simulink model "JenaFox_NCm"  (R2022a)
settings: Solver=VariableStepAuto  StartTime=0.0  StopTime=terminationConditions.stopTime  FixedStep=0.0001  MaxStep=solverParams.maxStep  RelTol=solverParams.relTol  AbsTol=solverParams.absTol
undefined symbols (not defined in the file): amplifier, c_coupling, d_coupling, g, GC, GM_h, IC, IC_v, motorHip, motorKnee, mu, offset, prop_const, smiData, terminationConditions, v, X, Y, Z
libraries: sm_lib x51, nesl_utility x46, simulink x23, simulink_extras x12, dspswit3 x2
(part 3 of 4)

== system JenaFox_NCm/JenaFox Model/Knee_r ==
  Right torque : Inport
  PS-Simulink Converter1 : nesl_utility/PS-Simulink Converter  PhysicalDomain=network_engine_domain  SubClassName=ps_output  LeftPortType=input  RightPortType=output  PseudoPeriodic=off  Frequencies=[]  VectorFormat=1-D array  Unit=1  AffineConversion=off
      settings: SourceProductBaseCode=SS,PW,VE
  PS-Simulink Converter2 : nesl_utility/PS-Simulink Converter  PhysicalDomain=network_engine_domain  SubClassName=ps_output  LeftPortType=input  RightPortType=output  PseudoPeriodic=off  Frequencies=[]  VectorFormat=1-D array  Unit=1  AffineConversion=off
      settings: SourceProductBaseCode=SS,PW,VE
  PS-Simulink Converter3 : nesl_utility/PS-Simulink Converter  PhysicalDomain=network_engine_domain  SubClassName=ps_output  LeftPortType=input  RightPortType=output  PseudoPeriodic=off  Frequencies=[]  VectorFormat=1-D array  Unit=1  AffineConversion=off
      settings: SourceProductBaseCode=SS,PW,VE
  Simulink-PS Converter : nesl_utility/Simulink-PS Converter  PhysicalDomain=network_engine_domain  SubClassName=ps_input  LeftPortType=input  RightPortType=output  PseudoPeriodic=off  Frequencies=[]  NoiseDistribution=none  NoiseParameters=[]  Unit=1  AffineConversion=off  FilteringAndDerivatives=provide  SimscapeFilterOrder=1  InputFilterTimeConstant=0.001  UdotUserProvided=0
      settings: SourceProductBaseCode=SS,PW,VE
  knee_r : sm_lib/Joints/Revolute Joint  JointMode=Normal  SenseConstraintForce=off  SenseConstraintForceX=off  SenseConstraintForceY=off  SenseConstraintForceZ=off  SenseConstraintTorque=off  SenseConstraintTorqueX=off  SenseConstraintTorqueY=off  SenseConstraintTorqueZ=off  SenseTotalForce=off  SenseTotalForceX=off  SenseTotalForceY=off  SenseTotalForceZ=off  SenseTotalTorque=off  SenseTotalTorqueX=off  SenseTotalTorqueY=off  SenseTotalTorqueZ=off  CompositeWrenchDir=FollowerOnBase  CompositeWrenchFrame=BaseFrame  EquilibriumPosition=0  EquilibriumPositionUnits=rad  SpringStiffness=0  SpringStiffnessUnits=N*m/rad  DampingCoefficient=d_joint  DampingCoefficientUnits=N*m/(rad/s)  TorqueActuationMode=InputTorque  MotionActuationMode=ComputedMotion  SensePosition=on  SenseVelocity=on  SenseAcceleration=on  SenseTorqueForce=off  SenseLowerLimitTorqueForce=off  SenseUpperLimitTorqueForce=off  LowerLimitSpecify=on  LowerLimitBound=IC.limit.phi_knee  LowerLimitBoundUnits=rad  LowerLimitStiffness=c_hs  LowerLimitStiffnessUnits=N*m/deg  LowerLimitDamping=d_hs  LowerLimitDampingUnits=N*m/(deg/s)  LowerLimitTransitionRegionWidth=0.1  LowerLimitTransitionRegionWidthUnits=deg  UpperLimitSpecify=on  UpperLimitBound=0  UpperLimitBoundUnits=rad  UpperLimitStiffness=c_hs  UpperLimitStiffnessUnits=N*m/deg  UpperLimitDamping=d_hs  UpperLimitDampingUnits=N*m/(deg/s)  UpperLimitTransitionRegionWidth=0.1  UpperLimitTransitionRegionWidthUnits=deg  PositionTargetSpecify=on  PositionTargetPriority=High  PositionTargetValue=IC.phi.knee_r  PositionTargetValueUnits=rad  VelocityTargetSpecify=on  VelocityTargetPriority=High  VelocityTargetValue=IC.vphi.knee_r  VelocityTargetValueUnits=rad/s
  Thigh : PMIOPort  Side=Left
  Shank : PMIOPort  Port=2  Side=Right
  tag scope: aphi_knee_r=global, phi_knee_r=global, vphi_knee_r=global
  wires:
  Right torque/1 -> Simulink-PS Converter/1  "torque servo right"
  PS-Simulink Converter2/1 -> [phi_knee_r]
  PS-Simulink Converter3/1 -> [aphi_knee_r]
  PS-Simulink Converter1/1 -> [vphi_knee_r]
  connections:
  Simulink-PS Converter/RConn1 -- knee_r/LConn2
  knee_r/RConn1 -- Shank/RConn1
  PS-Simulink Converter2/LConn1 -- knee_r/RConn2
  knee_r/RConn3 -- PS-Simulink Converter1/LConn1
  knee_r/LConn1 -- Thigh/RConn1
  PS-Simulink Converter3/LConn1 -- knee_r/RConn4

== system JenaFox_NCm/JenaFox Model/Shank_bottom_l ==
  Rigid Transform : sm_lib/Frames and Transforms/Rigid Transform  TranslationMethod=None  TranslationStandardOffset=0  TranslationLengthUnit=m  TranslationStandardAxis=+Z  TranslationCartesianOffset=[0 0 0]  TranslationROffset=0  TranslationROffsetUnits=m  TranslationZOffset=0  TranslationZOffsetUnits=m  TranslationThetaOffset=0  TranslationThetaOffsetUnits=deg  RotationMethod=AlignedAxes  RotationAngleUnits=deg  RotationStandardAxis=+Z  RotationAngle=0.0  RotationArbitraryAxis=[0 0 1]  FollAlignAxisA=+X  BaseAlignAxisA=-X  FollAlignAxisB=+Z  BaseAlignAxisB=+Y  RotationSequenceAxes=FollowerAxes  RotationSequence=XYX  RotationSequenceAngles=[0 0 0]  RotationSequenceAnglesUnits=deg  RotationMatrix=[1 0 0; 0 1 0; 0 0 1]
  Solid : sm_lib/Body Elements/File Solid  ExtGeomFileName=shank_bottom_ipt_92530788.STEP  UnitType=FromFile  ExtGeomFileUnits=m  StepReaderType=OCC  ExportConvexHullGeometry=off  InertiaType=Custom  Mass=smiData.Solid(4).mass  MassUnits=kg  CenterOfMass=smiData.Solid(4).CoM  CenterOfMassUnits=mm  MomentsOfInertia=smiData.Solid(4).MoI  MomentsOfInertiaUnits=kg*mm^2  ProductsOfInertia=smiData.Solid(4).PoI  ProductsOfInertiaUnits=kg*mm^2  BasedOnType=Density  Density=1000  DensityUnits=kg/m^3  DoExposeReferenceFrame=on  SerializedFrames=<Frames><Frame><Id>Frame1</Id><Value><Name>ground_contact</Name><Origin><Source>GeometricFeature</Source><FeatureName>circular curve 105</FeatureName></Origin><PrimaryAxis><DefinedDirection>+Y</DefinedDirection><Source>ReferenceFrame</Source><SourceDirection>-Y</SourceDirection><FeatureName></FeatureName></PrimaryAxis><SecondaryAxis><DefinedDirection>+X</DefinedDirection><Source>ReferenceFrame</Source><SourceDirection>+X</SourceDirection><FeatureName></FeatureName></SecondaryAxis></Value></Frame><Frame><Id>Frame2</Id><Value><Name>spring_bottom</Name><Origin><Source>GeometricFeature</Source><FeatureName>circular curve 81</FeatureName></Origin><PrimaryAxis><DefinedDirection>+Y</DefinedDirection><Source>ReferenceFrame</Source><SourceDirection>-Y</SourceDirection><FeatureName></FeatureName></PrimaryAxis><SecondaryAxis><DefinedDirection>+X</DefinedDirection><Source>ReferenceFrame</Source><SourceDirection>+X</SourceDirection><FeatureName></FeatureName></SecondaryAxis></Value></Frame></Frames>  GraphicType=FromGeometry  MarkerShape=Sphere  MarkerSize=10  GraphicVisPropType=SimpleVisualProperties  GraphicDiffuseColor=smiData.Solid(4).color  GraphicSpecularColor=[0.5 0.5 0.5 1.0]  GraphicAmbientColor=[0.15 0.15 0.15 1.0]  GraphicEmissiveColor=[0.0 0.0 0.0 1.0]  GraphicShininess=75  GraphicOpacity=smiData.Solid(4).opacity
  Linear elastic joint : PMIOPort  Side=Left
  Toe : PMIOPort  Port=2  Side=Right
  connections:
  Toe/RConn1 -- Solid/LConn1
  Rigid Transform/RConn1 -- Linear elastic joint/RConn1
  Rigid Transform/LConn1 -- Solid/LConn2

== system JenaFox_NCm/JenaFox Model/Shank_bottom_r ==
  Rigid Transform : sm_lib/Frames and Transforms/Rigid Transform  TranslationMethod=None  TranslationStandardOffset=0  TranslationLengthUnit=m  TranslationStandardAxis=+Z  TranslationCartesianOffset=[0 0 0]  TranslationROffset=0  TranslationROffsetUnits=m  TranslationZOffset=0  TranslationZOffsetUnits=m  TranslationThetaOffset=0  TranslationThetaOffsetUnits=deg  RotationMethod=AlignedAxes  RotationAngleUnits=deg  RotationStandardAxis=+Z  RotationAngle=0.0  RotationArbitraryAxis=[0 0 1]  FollAlignAxisA=+X  BaseAlignAxisA=+X  FollAlignAxisB=+Z  BaseAlignAxisB=+Y  RotationSequenceAxes=FollowerAxes  RotationSequence=XYX  RotationSequenceAngles=[0 0 0]  RotationSequenceAnglesUnits=deg  RotationMatrix=[1 0 0; 0 1 0; 0 0 1]
  Solid : sm_lib/Body Elements/File Solid  ExtGeomFileName=shank_bottom_ipt_92530788.STEP  UnitType=FromFile  ExtGeomFileUnits=m  StepReaderType=OCC  ExportConvexHullGeometry=off  InertiaType=Custom  Mass=smiData.Solid(4).mass  MassUnits=kg  CenterOfMass=smiData.Solid(4).CoM  CenterOfMassUnits=mm  MomentsOfInertia=smiData.Solid(4).MoI  MomentsOfInertiaUnits=kg*mm^2  ProductsOfInertia=smiData.Solid(4).PoI  ProductsOfInertiaUnits=kg*mm^2  BasedOnType=Density  Density=1000  DensityUnits=kg/m^3  DoExposeReferenceFrame=off  SerializedFrames=<Frames><Frame><Id>Frame1</Id><Value><Name>ground_contact</Name><Origin><Source>GeometricFeature</Source><FeatureName>circular curve 105</FeatureName></Origin><PrimaryAxis><DefinedDirection>+Y</DefinedDirection><Source>ReferenceFrame</Source><SourceDirection>-Y</SourceDirection><FeatureName></FeatureName></PrimaryAxis><SecondaryAxis><DefinedDirection>+X</DefinedDirection><Source>ReferenceFrame</Source><SourceDirection>+X</SourceDirection><FeatureName></FeatureName></SecondaryAxis></Value></Frame><Frame><Id>Frame2</Id><Value><Name>spring_bottom</Name><Origin><Source>GeometricFeature</Source><FeatureName>circular curve 81</FeatureName></Origin><PrimaryAxis><DefinedDirection>+Y</DefinedDirection><Source>ReferenceFrame</Source><SourceDirection>-Y</SourceDirection><FeatureName></FeatureName></PrimaryAxis><SecondaryAxis><DefinedDirection>+X</DefinedDirection><Source>ReferenceFrame</Source><SourceDirection>+X</SourceDirection><FeatureName></FeatureName></SecondaryAxis></Value></Frame></Frames>  GraphicType=FromGeometry  MarkerShape=Sphere  MarkerSize=10  GraphicVisPropType=SimpleVisualProperties  GraphicDiffuseColor=smiData.Solid(4).color  GraphicSpecularColor=[0.5 0.5 0.5 1.0]  GraphicAmbientColor=[0.15 0.15 0.15 1.0]  GraphicEmissiveColor=[0.0 0.0 0.0 1.0]  GraphicShininess=75  GraphicOpacity=smiData.Solid(4).opacity
  Linear elastic joint : PMIOPort  Side=Left
  Toe : PMIOPort  Port=2  Side=Right
  connections:
  Toe/RConn1 -- Solid/LConn1
  Rigid Transform/RConn1 -- Linear elastic joint/RConn1
  Rigid Transform/LConn1 -- Solid/RConn1

== system JenaFox_NCm/JenaFox Model/Shank_top_l ==
  Rigid Transform : sm_lib/Frames and Transforms/Rigid Transform  TranslationMethod=StandardAxis  TranslationStandardOffset=springAnkle.rl_l  TranslationLengthUnit=m  TranslationStandardAxis=+Z  TranslationCartesianOffset=[0 0 0]  TranslationROffset=0  TranslationROffsetUnits=m  TranslationZOffset=0  TranslationZOffsetUnits=m  TranslationThetaOffset=0  TranslationThetaOffsetUnits=deg  RotationMethod=AlignedAxes  RotationAngleUnits=deg  RotationStandardAxis=+Z  RotationAngle=0.0  RotationArbitraryAxis=[0 0 1]  FollAlignAxisA=+X  BaseAlignAxisA=+X  FollAlignAxisB=+Y  BaseAlignAxisB=+Z  RotationSequenceAxes=FollowerAxes  RotationSequence=XYX  RotationSequenceAngles=[0 0 0]  RotationSequenceAnglesUnits=deg  RotationMatrix=[1 0 0; 0 1 0; 0 0 1]
  Solid : sm_lib/Body Elements/File Solid  ExtGeomFileName=shank_top_ipt_5be12039.STEP  UnitType=FromFile  ExtGeomFileUnits=m  StepReaderType=OCC  ExportConvexHullGeometry=off  InertiaType=Custom  Mass=smiData.Solid(3).mass  MassUnits=kg  CenterOfMass=smiData.Solid(3).CoM  CenterOfMassUnits=mm  MomentsOfInertia=smiData.Solid(3).MoI  MomentsOfInertiaUnits=kg*mm^2  ProductsOfInertia=smiData.Solid(3).PoI  ProductsOfInertiaUnits=kg*mm^2  BasedOnType=Density  Density=1000  DensityUnits=kg/m^3  DoExposeReferenceFrame=off  SerializedFrames=<Frames><Frame><Id>Frame1</Id><Value><Name>spring_top</Name><Origin><Source>GeometricFeature</Source><FeatureName>circular curve 166</FeatureName></Origin><PrimaryAxis><DefinedDirection>+Y</DefinedDirection><Source>ReferenceFrame</Source><SourceDirection>-Y</SourceDirection><FeatureName></FeatureName></PrimaryAxis><SecondaryAxis><DefinedDirection>+X</DefinedDirection><Source>GeometricFeature</Source><SourceDirection>+X</SourceDirection><FeatureName>segment 110</FeatureName></SecondaryAxis></Value></Frame><Frame><Id>Frame2</Id><Value><Name>knee</Name><Origin><Source>GeometricFeature</Source><FeatureName>circular curve 135</FeatureName></Origin><PrimaryAxis><DefinedDirection>-X</DefinedDirection><Source>GeometricFeature</Source><SourceDirection>+Z</SourceDirection><FeatureName>segment 80</FeatureName></PrimaryAxis><SecondaryAxis><DefinedDirection>+Y</DefinedDirection><Source>GeometricFeature</Source><SourceDirection>+X</SourceDirection><FeatureName>segment 115</FeatureName></SecondaryAxis></Value></Frame></Frames>  GraphicType=FromGeometry  MarkerShape=Sphere  MarkerSize=10  GraphicVisPropType=SimpleVisualProperties  GraphicDiffuseColor=smiData.Solid(3).color  GraphicSpecularColor=[0.5 0.5 0.5 1.0]  GraphicAmbientColor=[0.15 0.15 0.15 1.0]  GraphicEmissiveColor=[0.0 0.0 0.0 1.0]  GraphicShininess=75  GraphicOpacity=smiData.Solid(3).opacity
  Knee : PMIOPort  Side=Left
  Linear joint : PMIOPort  Port=2  Side=Right
  connections:
  Knee/RConn1 -- Solid/RConn1
  Rigid Transform/RConn1 -- Solid/LConn1
  Linear joint/RConn1 -- Rigid Transform/LConn1

== system JenaFox_NCm/JenaFox Model/Shank_top_r ==
  Rigid Transform : sm_lib/Frames and Transforms/Rigid Transform  TranslationMethod=StandardAxis  TranslationStandardOffset=springAnkle.rl_r  TranslationLengthUnit=m  TranslationStandardAxis=+Z  TranslationCartesianOffset=[0 0 0]  TranslationROffset=0  TranslationROffsetUnits=m  TranslationZOffset=0  TranslationZOffsetUnits=m  TranslationThetaOffset=0  TranslationThetaOffsetUnits=deg  RotationMethod=AlignedAxes  RotationAngleUnits=deg  RotationStandardAxis=+Z  RotationAngle=0.0  RotationArbitraryAxis=[0 0 1]  FollAlignAxisA=+X  BaseAlignAxisA=+X  FollAlignAxisB=+Y  BaseAlignAxisB=+Z  RotationSequenceAxes=FollowerAxes  RotationSequence=XYX  RotationSequenceAngles=[0 0 0]  RotationSequenceAnglesUnits=deg  RotationMatrix=[1 0 0; 0 1 0; 0 0 1]
  Solid : sm_lib/Body Elements/File Solid  ExtGeomFileName=shank_top_ipt_5be12039.STEP  UnitType=FromFile  ExtGeomFileUnits=m  StepReaderType=OCC  ExportConvexHullGeometry=off  InertiaType=Custom  Mass=smiData.Solid(3).mass  MassUnits=kg  CenterOfMass=smiData.Solid(3).CoM  CenterOfMassUnits=mm  MomentsOfInertia=smiData.Solid(3).MoI  MomentsOfInertiaUnits=kg*mm^2  ProductsOfInertia=smiData.Solid(3).PoI  ProductsOfInertiaUnits=kg*mm^2  BasedOnType=Density  Density=1000  DensityUnits=kg/m^3  DoExposeReferenceFrame=off  SerializedFrames=<Frames><Frame><Id>Frame1</Id><Value><Name>spring_top</Name><Origin><Source>GeometricFeature</Source><FeatureName>circular curve 166</FeatureName></Origin><PrimaryAxis><DefinedDirection>+Y</DefinedDirection><Source>ReferenceFrame</Source><SourceDirection>-Y</SourceDirection><FeatureName></FeatureName></PrimaryAxis><SecondaryAxis><DefinedDirection>+X</DefinedDirection><Source>GeometricFeature</Source><SourceDirection>+X</SourceDirection><FeatureName>segment 110</FeatureName></SecondaryAxis></Value></Frame><Frame><Id>Frame2</Id><Value><Name>shank_knee_right</Name><Origin><Source>GeometricFeature</Source><FeatureName>circular curve 135</FeatureName></Origin><PrimaryAxis><DefinedDirection>+X</DefinedDirection><Source>GeometricFeature</Source><SourceDirection>+Z</SourceDirection><FeatureName>segment 110</FeatureName></PrimaryAxis><SecondaryAxis><DefinedDirection>+Y</DefinedDirection><Source>GeometricFeature</Source><SourceDirection>+X</SourceDirection><FeatureName>segment 138</FeatureName></SecondaryAxis></Value></Frame></Frames>  GraphicType=FromGeometry  MarkerShape=Sphere  MarkerSize=10  GraphicVisPropType=SimpleVisualProperties  GraphicDiffuseColor=smiData.Solid(3).color  GraphicSpecularColor=[0.5 0.5 0.5 1.0]  GraphicAmbientColor=[0.15 0.15 0.15 1.0]  GraphicEmissiveColor=[0.0 0.0 0.0 1.0]  GraphicShininess=75  GraphicOpacity=smiData.Solid(3).opacity
  Knee : PMIOPort  Side=Left
  Linear joint : PMIOPort  Port=2  Side=Right
  connections:
  Knee/RConn1 -- Solid/RConn1
  Rigid Transform/RConn1 -- Solid/LConn1
  Linear joint/RConn1 -- Rigid Transform/LConn1

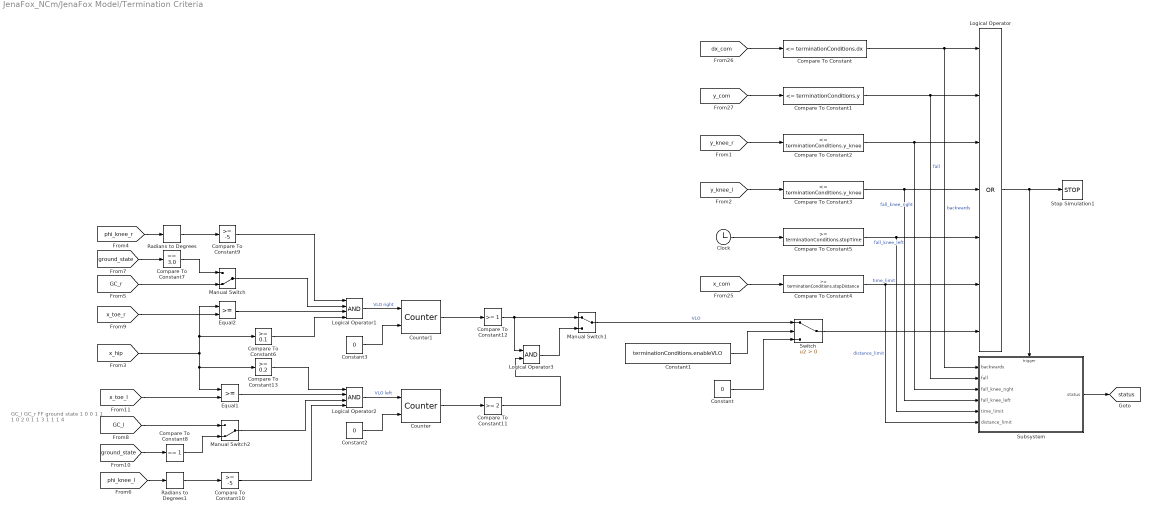
== system JenaFox_NCm/JenaFox Model/Termination Criteria ==
  note: GC_l   GC_r   FF   ground state
      | 1         0         0       1
      | 1         1         0       2
      | 0         1         1       3
      | 1         1         1       4
  Clock : Clock
  Compare To Constant : simulink/Logic and Bit Operations/Compare To Constant  relop=<=  const=terminationConditions.dx  OutDataTypeStr=boolean
  Compare To Constant1 : simulink/Logic and Bit Operations/Compare To Constant  relop=<=  const=terminationConditions.y  OutDataTypeStr=boolean
  Compare To Constant10 : simulink/Logic and Bit Operations/Compare To Constant  relop=>=  const=-5  OutDataTypeStr=boolean
  Compare To Constant11 : simulink/Logic and Bit Operations/Compare To Constant  relop=>=  const=2  OutDataTypeStr=boolean
  Compare To Constant12 : simulink/Logic and Bit Operations/Compare To Constant  relop=>=  const=1  OutDataTypeStr=boolean
  Compare To Constant13 : simulink/Logic and Bit Operations/Compare To Constant  relop=>=  const=0.2  OutDataTypeStr=boolean
  Compare To Constant2 : simulink/Logic and Bit Operations/Compare To Constant  relop=<=  const=terminationConditions.y_knee  OutDataTypeStr=boolean
  Compare To Constant3 : simulink/Logic and Bit Operations/Compare To Constant  relop=<=  const=terminationConditions.y_knee  OutDataTypeStr=boolean
  Compare To Constant4 : simulink/Logic and Bit Operations/Compare To Constant  relop=>=  const=terminationConditions.stopDistance  OutDataTypeStr=boolean
  Compare To Constant5 : simulink/Logic and Bit Operations/Compare To Constant  relop=>=  const=terminationConditions.stopTime  OutDataTypeStr=boolean
  Compare To Constant6 : simulink/Logic and Bit Operations/Compare To Constant  relop=>=  const=0.1  OutDataTypeStr=boolean
  Compare To Constant7 : simulink/Logic and Bit Operations/Compare To Constant  relop===  const=3.0  OutDataTypeStr=boolean
  Compare To Constant8 : simulink/Logic and Bit Operations/Compare To Constant  relop===  const=1  OutDataTypeStr=boolean
  Compare To Constant9 : simulink/Logic and Bit Operations/Compare To Constant  relop=>=  const=-5  OutDataTypeStr=boolean
  Constant : Constant  Value=0
  Constant1 : Constant  Value=terminationConditions.enableVLO
  Constant2 : Constant  Value=0
  Constant3 : Constant  Value=0
  Counter : dspswit3/Counter  Direction=Up  CountEvent=Rising edge  CounterSize=User defined  MaxCount=255  InitialCount=0  Output=Count  HitValue=32  ResetInput=on  SamplesPerFrame=1  Ts=1  CntDtype=double  HitDtype=Logical
  Counter1 : dspswit3/Counter  Direction=Up  CountEvent=Rising edge  CounterSize=User defined  MaxCount=255  InitialCount=0  Output=Count  HitValue=32  ResetInput=on  SamplesPerFrame=1  Ts=1  CntDtype=double  HitDtype=Logical
  Equal1 : RelationalOperator  OutDataTypeStr=boolean  RndMeth=Simplest  InputSameDT=off
  Equal2 : RelationalOperator  OutDataTypeStr=boolean  RndMeth=Simplest  InputSameDT=off
  Logical Operator : Logic  Operator=OR  Inputs=7  AllPortsSameDT=off  OutDataTypeStr=boolean
  Logical Operator1 : Logic  Inputs=4  AllPortsSameDT=off  OutDataTypeStr=boolean
  Logical Operator2 : Logic  Inputs=4  AllPortsSameDT=off  OutDataTypeStr=boolean
  Logical Operator3 : Logic  AllPortsSameDT=off  OutDataTypeStr=boolean
  Manual Switch : ManualSwitch  CurrentSetting=0
  Manual Switch1 : ManualSwitch
  Manual Switch2 : ManualSwitch  CurrentSetting=0
  Radians to Degrees : simulink_extras/Transformations/Radians to Degrees
  Radians to Degrees1 : simulink_extras/Transformations/Radians to Degrees
  Stop Simulation1 : Stop
  Subsystem : Subsystem
  Switch : Switch  Criteria=u2 > Threshold  SaturateOnIntegerOverflow=off  InputSameDT=off
  tag scope: status=global
  wires:
  [y_knee_r] -> Compare To Constant2/1
  [y_knee_l] -> Compare To Constant3/1
  Clock/1 -> Compare To Constant5/1
  Compare To Constant5/1 -> Subsystem/5(time_limit), Logical Operator/5  "time_limit"
  Compare To Constant/1 -> Subsystem/1(backwards), Logical Operator/1  "backwards"
  Compare To Constant1/1 -> Subsystem/2(fall), Logical Operator/2  "fall"
  Compare To Constant2/1 -> Subsystem/3(fall_knee_right), Logical Operator/3  "fall_knee_right"
  Compare To Constant3/1 -> Subsystem/4(fall_knee_left), Logical Operator/4  "fall_knee_left"
  Subsystem/1(status) -> [status]
  [y_com] -> Compare To Constant1/1
  [dx_com] -> Compare To Constant/1
  [x_com] -> Compare To Constant4/1
  Compare To Constant4/1 -> Subsystem/6(distance_limit), Logical Operator/6  "distance_limit"
  Logical Operator/1 -> Stop Simulation1/1, Subsystem/Trigger
  [ground_state] -> Compare To Constant7/1
  [ground_state] -> Compare To Constant8/1
  [GC_r] -> Manual Switch/2
  Compare To Constant7/1 -> Manual Switch/1
  [x_hip] -> Equal2/1, Compare To Constant6/1, Equal1/1, Compare To Constant13/1
  [GC_l] -> Manual Switch2/1
  Compare To Constant8/1 -> Manual Switch2/2
  Logical Operator2/1 -> Counter/1  "VLO left"
  [x_toe_l] -> Equal1/2
  [x_toe_r] -> Equal2/2
  Compare To Constant6/1 -> Logical Operator1/4
  Equal1/1 -> Logical Operator2/2
  Manual Switch2/1 -> Logical Operator2/3
  Constant/1 -> Switch/3
  Constant1/1 -> Switch/2
  Switch/1 -> Logical Operator/7
  Manual Switch1/1 -> Switch/1  "VLO"
  [phi_knee_r] -> Radians to Degrees/1
  Equal2/1 -> Logical Operator1/3
  Manual Switch/1 -> Logical Operator1/2
  Compare To Constant9/1 -> Logical Operator1/1
  Radians to Degrees/1 -> Compare To Constant9/1
  [phi_knee_l] -> Radians to Degrees1/1
  Radians to Degrees1/1 -> Compare To Constant10/1
  Compare To Constant10/1 -> Logical Operator2/4
  Constant2/1 -> Counter/2
  Counter/1 -> Compare To Constant11/1
  Compare To Constant11/1 -> Logical Operator3/2
  Logical Operator1/1 -> Counter1/1  "VLO right"
  Constant3/1 -> Counter1/2
  Counter1/1 -> Compare To Constant12/1
  Compare To Constant12/1 -> Logical Operator3/1, Manual Switch1/1
  Logical Operator3/1 -> Manual Switch1/2
  Compare To Constant13/1 -> Logical Operator2/1

== system JenaFox_NCm/JenaFox Model/Thigh_l ==
  Solid : sm_lib/Body Elements/File Solid  ExtGeomFileName=thigh_left_ipt_d01cdd9b.STEP  UnitType=FromFile  ExtGeomFileUnits=m  StepReaderType=OCC  ExportConvexHullGeometry=off  InertiaType=Custom  Mass=smiData.Solid(2).mass  MassUnits=kg  CenterOfMass=smiData.Solid(2).CoM  CenterOfMassUnits=mm  MomentsOfInertia=smiData.Solid(2).MoI  MomentsOfInertiaUnits=kg*mm^2  ProductsOfInertia=smiData.Solid(2).PoI  ProductsOfInertiaUnits=kg*mm^2  BasedOnType=Density  Density=1000  DensityUnits=kg/m^3  DoExposeReferenceFrame=off  SerializedFrames=<Frames><Frame><Id>Frame1</Id><Value><Name>thigh_left_knee</Name><Origin><Source>GeometricFeature</Source><FeatureName>planar surface 172</FeatureName></Origin><PrimaryAxis><DefinedDirection>+Z</DefinedDirection><Source>ReferenceFrame</Source><SourceDirection>-Y</SourceDirection><FeatureName></FeatureName></PrimaryAxis><SecondaryAxis><DefinedDirection>+X</DefinedDirection><Source>ReferenceFrame</Source><SourceDirection>+X</SourceDirection><FeatureName></FeatureName></SecondaryAxis></Value></Frame><Frame><Id>Frame2</Id><Value><Name>thigh_left_hip</Name><Origin><Source>GeometricFeature</Source><FeatureName>circular curve 156</FeatureName></Origin><PrimaryAxis><DefinedDirection>+Z</DefinedDirection><Source>ReferenceFrame</Source><SourceDirection>-Y</SourceDirection><FeatureName></FeatureName></PrimaryAxis><SecondaryAxis><DefinedDirection>+X</DefinedDirection><Source>ReferenceFrame</Source><SourceDirection>+X</SourceDirection><FeatureName></FeatureName></SecondaryAxis></Value></Frame></Frames>  GraphicType=FromGeometry  MarkerShape=Sphere  MarkerSize=10  GraphicVisPropType=SimpleVisualProperties  GraphicDiffuseColor=smiData.Solid(2).color  GraphicSpecularColor=[0.5 0.5 0.5 1.0]  GraphicAmbientColor=[0.15 0.15 0.15 1.0]  GraphicEmissiveColor=[0.0 0.0 0.0 1.0]  GraphicShininess=75  GraphicOpacity=smiData.Solid(2).opacity
  Hip : PMIOPort  Side=Left
  Knee : PMIOPort  Port=2  Side=Right
  connections:
  Hip/RConn1 -- Solid/RConn1
  Knee/RConn1 -- Solid/LConn1

== system JenaFox_NCm/JenaFox Model/Thigh_r ==
  Solid : sm_lib/Body Elements/File Solid  ExtGeomFileName=thigh_left_ipt_d01cdd9b.STEP  UnitType=FromFile  ExtGeomFileUnits=m  StepReaderType=OCC  ExportConvexHullGeometry=off  InertiaType=Custom  Mass=smiData.Solid(2).mass  MassUnits=kg  CenterOfMass=smiData.Solid(2).CoM  CenterOfMassUnits=mm  MomentsOfInertia=smiData.Solid(2).MoI  MomentsOfInertiaUnits=kg*mm^2  ProductsOfInertia=smiData.Solid(2).PoI  ProductsOfInertiaUnits=kg*mm^2  BasedOnType=Density  Density=1000  DensityUnits=kg/m^3  DoExposeReferenceFrame=off  SerializedFrames=<Frames><Frame><Id>Frame1</Id><Value><Name>thigh_right_knee</Name><Origin><Source>GeometricFeature</Source><FeatureName>circular curve 616</FeatureName></Origin><PrimaryAxis><DefinedDirection>+Z</DefinedDirection><Source>ReferenceFrame</Source><SourceDirection>+Y</SourceDirection><FeatureName></FeatureName></PrimaryAxis><SecondaryAxis><DefinedDirection>+X</DefinedDirection><Source>ReferenceFrame</Source><SourceDirection>-X</SourceDirection><FeatureName></FeatureName></SecondaryAxis></Value></Frame><Frame><Id>Frame2</Id><Value><Name>thigh_right_hip</Name><Origin><Source>GeometricFeature</Source><FeatureName>circular curve 280</FeatureName></Origin><PrimaryAxis><DefinedDirection>+Z</DefinedDirection><Source>ReferenceFrame</Source><SourceDirection>+Y</SourceDirection><FeatureName></FeatureName></PrimaryAxis><SecondaryAxis><DefinedDirection>+X</DefinedDirection><Source>ReferenceFrame</Source><SourceDirection>-X</SourceDirection><FeatureName></FeatureName></SecondaryAxis></Value></Frame></Frames>  GraphicType=FromGeometry  MarkerShape=Sphere  MarkerSize=10  GraphicVisPropType=SimpleVisualProperties  GraphicDiffuseColor=smiData.Solid(2).color  GraphicSpecularColor=[0.5 0.5 0.5 1.0]  GraphicAmbientColor=[0.15 0.15 0.15 1.0]  GraphicEmissiveColor=[0.0 0.0 0.0 1.0]  GraphicShininess=75  GraphicOpacity=smiData.Solid(2).opacity
  Hip : PMIOPort  Side=Left
  Knee : PMIOPort  Port=2  Side=Right
  connections:
  Knee/RConn1 -- Solid/LConn1
  Solid/RConn1 -- Hip/RConn1

== system JenaFox_NCm/JenaFox Model/Trunk ==
  Solid : sm_lib/Body Elements/File Solid  ExtGeomFileName=trunk_ipt_7785b5f2.STEP  UnitType=FromFile  ExtGeomFileUnits=m  StepReaderType=OCC  ExportConvexHullGeometry=off  InertiaType=Custom  Mass=smiData.Solid(1).mass  MassUnits=kg  CenterOfMass=smiData.Solid(1).CoM  CenterOfMassUnits=mm  MomentsOfInertia=smiData.Solid(1).MoI  MomentsOfInertiaUnits=kg*mm^2  ProductsOfInertia=smiData.Solid(1).PoI  ProductsOfInertiaUnits=kg*mm^2  BasedOnType=Density  Density=1000  DensityUnits=kg/m^3  DoExposeReferenceFrame=off  SerializedFrames=<Frames><Frame><Id>Frame1</Id><Value><Name>hip_right</Name><Origin><Source>GeometricFeature</Source><FeatureName>circular curve 591</FeatureName></Origin><PrimaryAxis><DefinedDirection>+Z</DefinedDirection><Source>ReferenceFrame</Source><SourceDirection>+X</SourceDirection><FeatureName></FeatureName></PrimaryAxis><SecondaryAxis><DefinedDirection>+X</DefinedDirection><Source>ReferenceFrame</Source><SourceDirection>-Z</SourceDirection><FeatureName></FeatureName></SecondaryAxis></Value></Frame><Frame><Id>Frame2</Id><Value><Name>hip_left</Name><Origin><Source>GeometricFeature</Source><FeatureName>circular curve 612</FeatureName></Origin><PrimaryAxis><DefinedDirection>+Z</DefinedDirection><Source>ReferenceFrame</Source><SourceDirection>+X</SourceDirection><FeatureName></FeatureName></PrimaryAxis><SecondaryAxis><DefinedDirection>+X</DefinedDirection><Source>ReferenceFrame</Source><SourceDirection>-Z</SourceDirection><FeatureName></FeatureName></SecondaryAxis></Value></Frame><Frame><Id>Frame3</Id><Value><Name>boom_connector</Name><Origin><Source>GeometricFeature</Source><FeatureName>circular curve 1475</FeatureName></Origin><PrimaryAxis><DefinedDirection>+X</DefinedDirection><Source>ReferenceFrame</Source><SourceDirection>-Z</SourceDirection><FeatureName></FeatureName></PrimaryAxis><SecondaryAxis><DefinedDirection>+Y</DefinedDirection><Source>ReferenceFrame</Source><SourceDirection>+Y</SourceDirection><FeatureName></FeatureName></SecondaryAxis></Value></Frame></Frames>  GraphicType=FromGeometry  MarkerShape=Sphere  MarkerSize=10  GraphicVisPropType=SimpleVisualProperties  GraphicDiffuseColor=smiData.Solid(1).color  GraphicSpecularColor=[0.5 0.5 0.5 1.0]  GraphicAmbientColor=[0.15 0.15 0.15 1.0]  GraphicEmissiveColor=[0.0 0.0 0.0 1.0]  GraphicShininess=75  GraphicOpacity=smiData.Solid(1).opacity
  Hip left : PMIOPort  Side=Right
  Hip right : PMIOPort  Port=2  Side=Right
  Boom : PMIOPort  Port=3  Side=Left
  connections:
  Solid/RConn1 -- Hip left/RConn1
  Hip right/RConn1 -- Solid/LConn1
  Boom/RConn1 -- Solid/LConn2

== system JenaFox_NCm/Motor Model/hip_motor_left ==
  note: IC_phi_motor
  note: IC_v_motor
  note: due to neglectible inductivity the
      | PT1 - transfer function is reduced to an
      | proportional transfer function
      | (Modellbildung und Simulation dynamischer Systeme, S.122)
  U : Inport
  phi_motor : Inport  Port=2
  Add1 : Sum  Inputs=+--
  M_func_hip1 : Lookup  InputValues=[-10^10 -motorHip.na -0.001 0 0.001 motorHip.na 10^10]  Table=[-motorHip.Mrg -motorHip.Mrg -motorHip.Mrhg 0 motorHip.Mrhg motorHip.Mrg motorHip.Mrg]  SaturateOnIntegerOverflow=off
  Radians to Degrees : simulink_extras/Transformations/Radians to Degrees
  Sum1 : Sum  Inputs=|+-
  elastic coupling : Sum  Inputs=+-
  elasticity : Gain  Gain=c_coupling.hip
  gearhead : Gain  Gain=motorHip.i
  gearhead1 : Gain  Gain=motorHip.i
  motor constant 1 : Gain  Gain=motorHip.k
  motor constant1 : Gain  Gain=motorHip.k
  motor interia : Gain  Gain=1/motorHip.Jm
  position : Integrator  InitialCondition=IC.motor.hip_l  ContinuousStateAttributes='position_hip'
  rotor resistor1 : Gain  Gain=1/motorHip.Ra
  speed : Integrator  InitialCondition=IC_v.motorHip  ContinuousStateAttributes='speed_hip'
  motor_torque : Outport  VectorParamsAs1DForOutWhenUnconnected=off
  current : Outport  Port=2  VectorParamsAs1DForOutWhenUnconnected=off
  wires:
  elasticity/1 -> motor_torque/1, gearhead1/1  "coupling torque"
  gearhead1/1 -> Add1/3
  phi_motor/1 -> elastic coupling/2
  U/1 -> Sum1/1
  Radians to Degrees/1 -> gearhead/1  "position in °"
  gearhead/1 -> elastic coupling/1
  elastic coupling/1 -> elasticity/1
  position/1 -> Radians to Degrees/1  "position"
  motor constant 1/1 -> Sum1/2  "inductive voltage"
  speed/1 -> motor constant 1/1, M_func_hip1/1, position/1  "motor speed"
  Sum1/1 -> rotor resistor1/1
  motor interia/1 -> speed/1  "acceleration"
  Add1/1 -> motor interia/1
  M_func_hip1/1 -> Add1/2  "friction torque"
  motor constant1/1 -> Add1/1  "motor torque"
  rotor resistor1/1 -> current/1, motor constant1/1  "current"

== system JenaFox_NCm/Motor Model/hip_motor_right ==
  note: IC_phi_motor
  note: IC_v_motor
  note: due to neglectible inductivity the
      | PT1 - transfer function is reduced to an
      | proportional transfer function
      | (Modellbildung und Simulation dynamischer Systeme, S.122)
  U : Inport
  phi_motor : Inport  Port=2
  Add1 : Sum  Inputs=+--
  M_func_hip1 : Lookup  InputValues=[-10^10 -motorHip.na -0.001 0 0.001 motorHip.na 10^10]  Table=[-motorHip.Mrg -motorHip.Mrg -motorHip.Mrhg 0 motorHip.Mrhg motorHip.Mrg motorHip.Mrg]  SaturateOnIntegerOverflow=off
  Radians to Degrees : simulink_extras/Transformations/Radians to Degrees
  Sum1 : Sum  Inputs=|+-
  elastic coupling : Sum  Inputs=+-
  elasticity : Gain  Gain=c_coupling.hip
  gearhead : Gain  Gain=motorHip.i
  gearhead1 : Gain  Gain=motorHip.i
  motor constant 1 : Gain  Gain=motorHip.k
  motor constant1 : Gain  Gain=motorHip.k
  motor interia : Gain  Gain=1/motorHip.Jm
  position : Integrator  InitialCondition=IC.motor.hip_r  ContinuousStateAttributes='position_hip'
  rotor resistor1 : Gain  Gain=1/motorHip.Ra
  speed : Integrator  InitialCondition=IC_v.motorHip  ContinuousStateAttributes='speed_hip'
  motor_torque : Outport  VectorParamsAs1DForOutWhenUnconnected=off
  current : Outport  Port=2  VectorParamsAs1DForOutWhenUnconnected=off
  wires:
  elasticity/1 -> motor_torque/1, gearhead1/1  "coupling torque"
  gearhead1/1 -> Add1/3
  phi_motor/1 -> elastic coupling/2
  U/1 -> Sum1/1
  Radians to Degrees/1 -> gearhead/1  "position in °"
  gearhead/1 -> elastic coupling/1
  elastic coupling/1 -> elasticity/1
  position/1 -> Radians to Degrees/1  "position"
  motor constant 1/1 -> Sum1/2  "inductive voltage"
  speed/1 -> motor constant 1/1, M_func_hip1/1, position/1  "motor speed"
  Sum1/1 -> rotor resistor1/1
  motor interia/1 -> speed/1  "acceleration"
  Add1/1 -> motor interia/1
  M_func_hip1/1 -> Add1/2  "friction torque"
  motor constant1/1 -> Add1/1  "motor torque"
  rotor resistor1/1 -> current/1, motor constant1/1  "current"

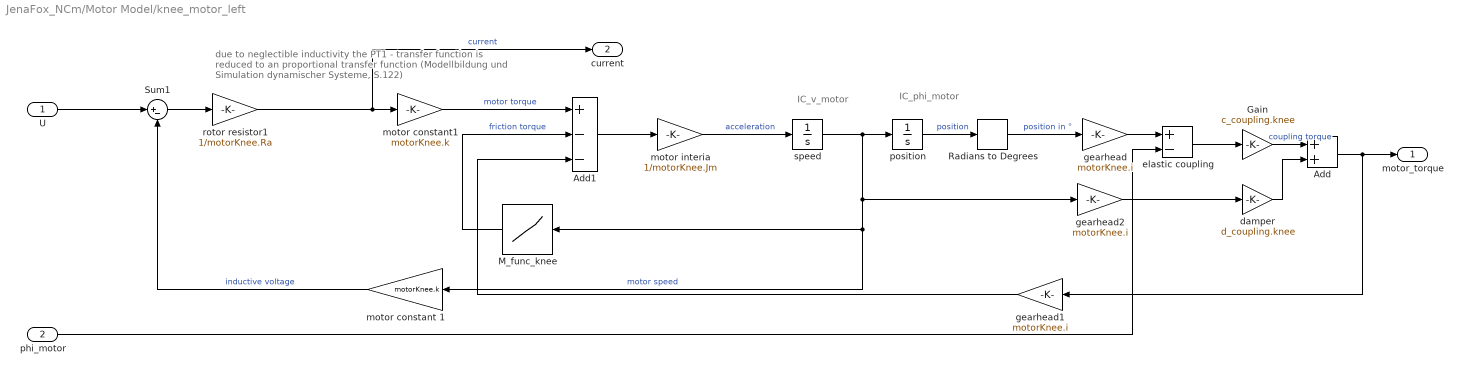
== system JenaFox_NCm/Motor Model/knee_motor_left ==
  note: due to neglectible inductivity the
      | PT1 - transfer function is reduced to an
      | proportional transfer function
      | (Modellbildung und Simulation dynamischer Systeme, S.122)
  note: IC_v_motor
  note: IC_phi_motor
  U : Inport
  phi_motor : Inport  Port=2
  Add : Sum
  Add1 : Sum  Inputs=+--
  Gain : Gain  Gain=c_coupling.knee
  M_func_knee : Lookup  InputValues=[-10^10 -motorKnee.na -0.001 0 0.001 motorKnee.na 10^10]  Table=[-motorKnee.Mrg -motorKnee.Mrg -motorKnee.Mrhg 0 motorKnee.Mrhg motorKnee.Mrg motorKnee.Mrg]  SaturateOnIntegerOverflow=off
  Radians to Degrees : simulink_extras/Transformations/Radians to Degrees
  Sum1 : Sum  Inputs=|+-
  damper : Gain  Gain=d_coupling.knee
  elastic coupling : Sum  Inputs=+-
  gearhead : Gain  Gain=motorKnee.i
  gearhead1 : Gain  Gain=motorKnee.i
  gearhead2 : Gain  Gain=motorKnee.i
  motor constant 1 : Gain  Gain=motorKnee.k
  motor constant1 : Gain  Gain=motorKnee.k
  motor interia : Gain  Gain=1/motorKnee.Jm
  position : Integrator  InitialCondition=IC.motor.knee_l  ContinuousStateAttributes='position_hip'
  rotor resistor1 : Gain  Gain=1/motorKnee.Ra
  speed : Integrator  InitialCondition=IC_v.motorKnee  ContinuousStateAttributes='speed_hip'
  motor_torque : Outport  VectorParamsAs1DForOutWhenUnconnected=off
  current : Outport  Port=2  VectorParamsAs1DForOutWhenUnconnected=off
  wires:
  gearhead1/1 -> Add1/3
  rotor resistor1/1 -> motor constant1/1, current/1  "current"
  motor constant1/1 -> Add1/1  "motor torque"
  M_func_knee/1 -> Add1/2  "friction torque"
  Add1/1 -> motor interia/1
  motor interia/1 -> speed/1  "acceleration"
  Sum1/1 -> rotor resistor1/1
  speed/1 -> position/1, M_func_knee/1, motor constant 1/1, gearhead2/1  "motor speed"
  position/1 -> Radians to Degrees/1  "position"
  elastic coupling/1 -> Gain/1
  gearhead/1 -> elastic coupling/1
  Radians to Degrees/1 -> gearhead/1  "position in °"
  U/1 -> Sum1/1
  phi_motor/1 -> elastic coupling/2
  motor constant 1/1 -> Sum1/2  "inductive voltage"
  Gain/1 -> Add/1  "coupling torque"
  Add/1 -> motor_torque/1, gearhead1/1
  gearhead2/1 -> damper/1
  damper/1 -> Add/2

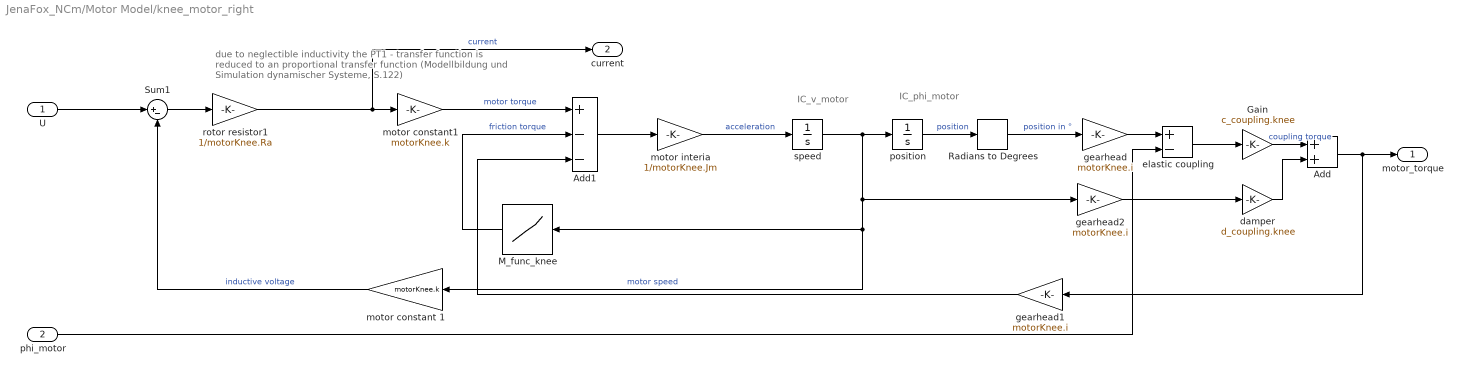
== system JenaFox_NCm/Motor Model/knee_motor_right ==
  note: due to neglectible inductivity the
      | PT1 - transfer function is reduced to an
      | proportional transfer function
      | (Modellbildung und Simulation dynamischer Systeme, S.122)
  note: IC_v_motor
  note: IC_phi_motor
  U : Inport
  phi_motor : Inport  Port=2
  Add : Sum
  Add1 : Sum  Inputs=+--
  Gain : Gain  Gain=c_coupling.knee
  M_func_knee : Lookup  InputValues=[-10^10 -motorKnee.na -0.001 0 0.001 motorKnee.na 10^10]  Table=[-motorKnee.Mrg -motorKnee.Mrg -motorKnee.Mrhg 0 motorKnee.Mrhg motorKnee.Mrg motorKnee.Mrg]  SaturateOnIntegerOverflow=off
  Radians to Degrees : simulink_extras/Transformations/Radians to Degrees
  Sum1 : Sum  Inputs=|+-
  damper : Gain  Gain=d_coupling.knee
  elastic coupling : Sum  Inputs=+-
  gearhead : Gain  Gain=motorKnee.i
  gearhead1 : Gain  Gain=motorKnee.i
  gearhead2 : Gain  Gain=motorKnee.i
  motor constant 1 : Gain  Gain=motorKnee.k
  motor constant1 : Gain  Gain=motorKnee.k
  motor interia : Gain  Gain=1/motorKnee.Jm
  position : Integrator  InitialCondition=IC.motor.knee_r  ContinuousStateAttributes='position_hip'
  rotor resistor1 : Gain  Gain=1/motorKnee.Ra
  speed : Integrator  InitialCondition=IC_v.motorKnee  ContinuousStateAttributes='speed_hip'
  motor_torque : Outport  VectorParamsAs1DForOutWhenUnconnected=off
  current : Outport  Port=2  VectorParamsAs1DForOutWhenUnconnected=off
  wires:
  gearhead1/1 -> Add1/3
  rotor resistor1/1 -> motor constant1/1, current/1  "current"
  motor constant1/1 -> Add1/1  "motor torque"
  M_func_knee/1 -> Add1/2  "friction torque"
  Add1/1 -> motor interia/1
  motor interia/1 -> speed/1  "acceleration"
  Sum1/1 -> rotor resistor1/1
  speed/1 -> position/1, M_func_knee/1, motor constant 1/1, gearhead2/1  "motor speed"
  position/1 -> Radians to Degrees/1  "position"
  elastic coupling/1 -> Gain/1
  gearhead/1 -> elastic coupling/1
  Radians to Degrees/1 -> gearhead/1  "position in °"
  U/1 -> Sum1/1
  phi_motor/1 -> elastic coupling/2
  motor constant 1/1 -> Sum1/2  "inductive voltage"
  Gain/1 -> Add/1  "coupling torque"
  Add/1 -> motor_torque/1, gearhead1/1
  gearhead2/1 -> damper/1
  damper/1 -> Add/2

== system JenaFox_NCm/Touchdown/Triggered Subsystem1 ==
  touchdown_in : Inport
  Trigger : TriggerPort  VariantControl=(inherit)
  touchdown_out : Outport
  wires:
  touchdown_in/1 -> touchdown_out/1

== system JenaFox_NCm/JenaFox Model/GCM Left/Ground Friction Model ==
  note: Horizontal Ground Friction Model
  note: Vertical Ground Stiction Model
  dy [m] : Inport
  vy [m/s] : Inport  Port=2
  x [m] : Inport  Port=3
  vx [m/s] : Inport  Port=4
  Contact! : EnablePort  StatesWhenEnabling=reset  PropagateVarSize=During execution
  Data Type Conversion : DataTypeConversion  OutDataTypeStr=double  SaturateOnIntegerOverflow=off  RndMeth=Floor
  Friction Switch : Subsystem
  Gain3 : Gain  Gain=GC.k_gy
  Gain4 : Gain  Gain=1/v.gy_max
  Logical Operator : Logic  Operator=NOT  AllPortsSameDT=off  OutDataTypeStr=boolean
  Mux1 : Mux  Inputs=2
  Sum1 : Sum
  X-Axis Kinetic Friction Model : Subsystem
  X-Axis Static Friction Model : Subsystem
  Y-Axis Ground Force : Fcn  Expr="- u(1)  *  (1-u(2)) * (u(2)<1)"
  Fy_Ground[N] : Outport  OutputWhenDisabled=reset  InitialOutput=0  VectorParamsAs1DForOutWhenUnconnected=off
      settings: AttributesFormatString=initial = '%<InitialOutput>'\nwhen disabled = '%<OutputWhenDisabled>'
  Fx_Friction [N] : Outport  Port=2  OutputWhenDisabled=reset  InitialOutput=0  VectorParamsAs1DForOutWhenUnconnected=off
      settings: AttributesFormatString=initial = '%<InitialOutput>'\nwhen\ndisabled\n'%<OutputWhenDisabled>'
  Stiction! : Outport  Port=3  OutputWhenDisabled=reset  InitialOutput=0  VectorParamsAs1DForOutWhenUnconnected=off
      settings: AttributesFormatString=initial = '%<InitialOutput>'\nwhen\ndisabled\n'%<OutputWhenDisabled>'
  wires:
  dy [m]/1 -> Gain3/1
  vy [m/s]/1 -> Gain4/1
  x [m]/1 -> X-Axis Static Friction Model/2(pos [m]), X-Axis Kinetic Friction Model/1(pos [m])
  vx [m/s]/1 -> X-Axis Static Friction Model/3(vel [m/s]), X-Axis Kinetic Friction Model/2(vel [m/s])
  X-Axis Kinetic Friction Model/1(posFP [m]) -> X-Axis Static Friction Model/4(posFP [m])
  X-Axis Kinetic Friction Model/3(F_Slide [N]) -> Sum1/2
  X-Axis Static Friction Model/1(F_Stick [N]) -> Sum1/1
  Sum1/1 -> Fx_Friction [N]/1
  Friction Switch/1(Stiction) -> X-Axis Static Friction Model/Enable, Logical Operator/1, Data Type Conversion/1
  X-Axis Static Friction Model/2(Sliding!) -> Friction Switch/1(Slide!)
  X-Axis Kinetic Friction Model/2(Stiction!) -> Friction Switch/2(Stick!)
  Logical Operator/1 -> X-Axis Kinetic Friction Model/Enable
  Data Type Conversion/1 -> Stiction!/1
  Mux1/1 -> Y-Axis Ground Force/1
  Gain3/1 -> Mux1/1
  Gain4/1 -> Mux1/2
  Y-Axis Ground Force/1 -> Fy_Ground[N]/1, X-Axis Static Friction Model/1(F_Normal [N]), X-Axis Kinetic Friction Model/3(F_Normal [N])

== system JenaFox_NCm/JenaFox Model/GCM Right/Ground Friction Model ==
  note: Horizontal Ground Friction Model
  note: Vertical Ground Stiction Model
  dy [m] : Inport
  vy [m/s] : Inport  Port=2
  x [m] : Inport  Port=3
  vx [m/s] : Inport  Port=4
  Contact! : EnablePort  StatesWhenEnabling=reset  PropagateVarSize=During execution
  Data Type Conversion : DataTypeConversion  OutDataTypeStr=double  SaturateOnIntegerOverflow=off  RndMeth=Floor
  Friction Switch : Subsystem
  Gain3 : Gain  Gain=GC.k_gy
  Gain4 : Gain  Gain=1/v.gy_max
  Logical Operator : Logic  Operator=NOT  AllPortsSameDT=off  OutDataTypeStr=boolean
  Mux1 : Mux  Inputs=2
  Sum1 : Sum
  X-Axis Kinetic Friction Model : Subsystem
  X-Axis Static Friction Model : Subsystem
  Y-Axis Ground Force : Fcn  Expr="- u(1)  *  (1-u(2)) * (u(2)<1)"
  Fy_Ground[N] : Outport  OutputWhenDisabled=reset  InitialOutput=0  VectorParamsAs1DForOutWhenUnconnected=off
      settings: AttributesFormatString=initial = '%<InitialOutput>'\nwhen disabled = '%<OutputWhenDisabled>'
  Fx_Friction [N] : Outport  Port=2  OutputWhenDisabled=reset  InitialOutput=0  VectorParamsAs1DForOutWhenUnconnected=off
      settings: AttributesFormatString=initial = '%<InitialOutput>'\nwhen\ndisabled\n'%<OutputWhenDisabled>'
  Stiction! : Outport  Port=3  OutputWhenDisabled=reset  InitialOutput=0  VectorParamsAs1DForOutWhenUnconnected=off
      settings: AttributesFormatString=initial = '%<InitialOutput>'\nwhen\ndisabled\n'%<OutputWhenDisabled>'
  wires:
  dy [m]/1 -> Gain3/1
  vy [m/s]/1 -> Gain4/1
  x [m]/1 -> X-Axis Static Friction Model/2(pos [m]), X-Axis Kinetic Friction Model/1(pos [m])
  vx [m/s]/1 -> X-Axis Static Friction Model/3(vel [m/s]), X-Axis Kinetic Friction Model/2(vel [m/s])
  X-Axis Kinetic Friction Model/1(posFP [m]) -> X-Axis Static Friction Model/4(posFP [m])
  X-Axis Kinetic Friction Model/3(F_Slide [N]) -> Sum1/2
  X-Axis Static Friction Model/1(F_Stick [N]) -> Sum1/1
  Sum1/1 -> Fx_Friction [N]/1
  Friction Switch/1(Stiction) -> X-Axis Static Friction Model/Enable, Logical Operator/1, Data Type Conversion/1
  X-Axis Static Friction Model/2(Sliding!) -> Friction Switch/1(Slide!)
  X-Axis Kinetic Friction Model/2(Stiction!) -> Friction Switch/2(Stick!)
  Logical Operator/1 -> X-Axis Kinetic Friction Model/Enable
  Data Type Conversion/1 -> Stiction!/1
  Mux1/1 -> Y-Axis Ground Force/1
  Gain3/1 -> Mux1/1
  Gain4/1 -> Mux1/2
  Y-Axis Ground Force/1 -> Fy_Ground[N]/1, X-Axis Static Friction Model/1(F_Normal [N]), X-Axis Kinetic Friction Model/3(F_Normal [N])

== system JenaFox_NCm/JenaFox Model/Ground Contact Model (GCM)/Starting time ==
  In1 : Inport
  Trigger : TriggerPort  VariantControl=(inherit)
  Out1 : Outport
  wires:
  In1/1 -> Out1/1

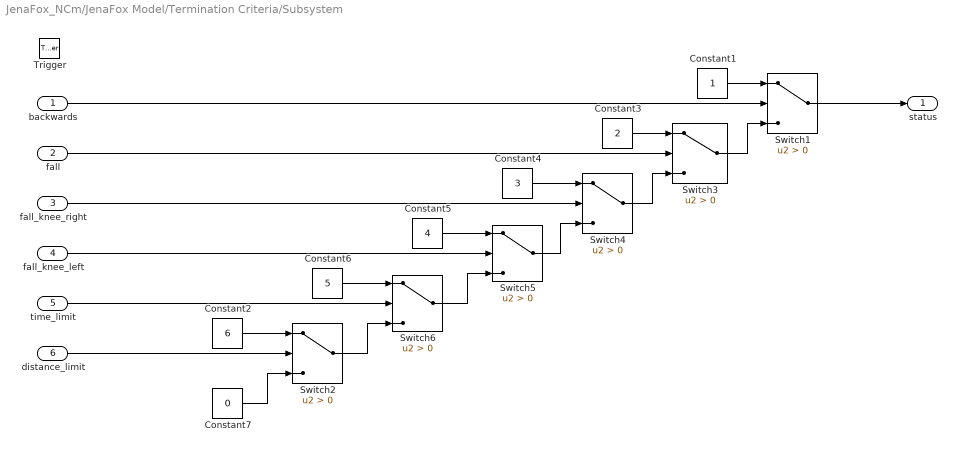
== system JenaFox_NCm/JenaFox Model/Termination Criteria/Subsystem ==
  backwards : Inport
  fall : Inport  Port=2
  fall_knee_right : Inport  Port=3
  fall_knee_left : Inport  Port=4
  time_limit : Inport  Port=5
  distance_limit : Inport  Port=6
  Trigger : TriggerPort  VariantControl=(inherit)  PortDimensions=1
  Constant1 : Constant
  Constant2 : Constant  Value=6
  Constant3 : Constant  Value=2
  Constant4 : Constant  Value=3
  Constant5 : Constant  Value=4
  Constant6 : Constant  Value=5
  Constant7 : Constant  Value=0
  Switch{1..6} (6 alike) : Switch  Criteria=u2 > Threshold  SaturateOnIntegerOverflow=off  InputSameDT=off
  status : Outport
  wires:
  backwards/1 -> Switch1/2
  Switch3/1 -> Switch1/3
  fall_knee_right/1 -> Switch4/2
  Switch4/1 -> Switch3/3
  fall_knee_left/1 -> Switch5/2
  Switch5/1 -> Switch4/3
  time_limit/1 -> Switch6/2
  Switch6/1 -> Switch5/3
  Constant1/1 -> Switch1/1
  Constant3/1 -> Switch3/1
  Constant4/1 -> Switch4/1
  Constant5/1 -> Switch5/1
  Constant6/1 -> Switch6/1
  Switch1/1 -> status/1
  Switch2/1 -> Switch6/3
  distance_limit/1 -> Switch2/2
  Constant2/1 -> Switch2/1
  fall/1 -> Switch3/2
  Constant7/1 -> Switch2/3

== system JenaFox_NCm/JenaFox Model/GCM Left/Ground Friction Model/Friction Switch ==
  note: Static/Kinetic Friction Switch
  Slide! : Inport
  Stick! : Inport  Port=2
  Memory : Memory
  S-R Flip-Flop : simulink_extras/Flip Flops/S-R Flip-Flop  initial_condition=1
  Terminator : Terminator
  Stiction : Outport  VectorParamsAs1DForOutWhenUnconnected=off
  wires:
  S-R Flip-Flop/1 -> Memory/1
  S-R Flip-Flop/2 -> Terminator/1
  Stick!/1 -> S-R Flip-Flop/1
  Slide!/1 -> S-R Flip-Flop/2
  Memory/1 -> Stiction/1

== system JenaFox_NCm/JenaFox Model/GCM Left/Ground Friction Model/X-Axis Kinetic Friction Model ==
  note: Kinetic Friction Model
  note: Footpoint Determiner
  note: Sliding Limit Detector
  pos [m] : Inport
  vel [m/s] : Inport  Port=2
  F_Normal [N] : Inport  Port=3
  Enable : EnablePort  StatesWhenEnabling=reset  PropagateVarSize=During execution
  Abs : Abs  SaturateOnIntegerOverflow=off
  Constant : Constant  Value=v.limit
  FixPt Relational Operator : RelationalOperator  Operator=>  OutDataTypeStr=boolean  ZeroCross=off  InputSameDT=off
  Memory : Memory  InheritSampleTime=on
  Negative : simulink/Logic and Bit Operations/Compare To Zero  relop=<  OutDataTypeStr=boolean
  Product : Product  RndMeth=Zero
  Sign1 : Signum
  Sum : Sum  Inputs=|+-
  reverse : Gain  Gain=-1
  sliding friction coefficient : Gain  Gain=mu.slide
  posFP [m] : Outport  VectorParamsAs1DForOutWhenUnconnected=off
      settings: AttributesFormatString=initial = '%<InitialOutput>'\nwhen disabled = '%<OutputWhenDisabled>'
  Stiction! : Outport  Port=2  OutputWhenDisabled=reset  InitialOutput=0  VectorParamsAs1DForOutWhenUnconnected=off
      settings: AttributesFormatString=initial = '%<InitialOutput>'\nwhen disabled = '%<OutputWhenDisabled>'
  F_Slide [N] : Outport  Port=3  OutputWhenDisabled=reset  InitialOutput=0  VectorParamsAs1DForOutWhenUnconnected=off
      settings: AttributesFormatString=initial = '%<InitialOutput>'\nwhen disabled = '%<OutputWhenDisabled>'
  wires:
  reverse/1 -> Product/1
  F_Normal [N]/1 -> sliding friction coefficient/1
  vel [m/s]/1 -> Sign1/1, Abs/1
  pos [m]/1 -> posFP [m]/1
  Product/1 -> F_Slide [N]/1
  sliding friction coefficient/1 -> Product/2
  Sign1/1 -> reverse/1
  Memory/1 -> FixPt Relational Operator/2
  Negative/1 -> Memory/1, FixPt Relational Operator/1
  Abs/1 -> Sum/1
  Sum/1 -> Negative/1
  Constant/1 -> Sum/2
  FixPt Relational Operator/1 -> Stiction!/1

== system JenaFox_NCm/JenaFox Model/GCM Left/Ground Friction Model/X-Axis Static Friction Model ==
  note: Stiction Limit Detector
  note: Static Friction Model
  note: Zero multiplication prevents
      | horizontal friction model from
      | oscillating between static and kinetic
      | friction when the vertical force is zero but
      | the ground level is not yet reached
      | in the upward motion
  F_Normal [N] : Inport
  pos [m] : Inport  Port=2
  vel [m/s] : Inport  Port=3
  posFP [m] : Inport  Port=4
  Enable : EnablePort  StatesWhenEnabling=reset  PropagateVarSize=During execution
  Abs : Abs  SaturateOnIntegerOverflow=off
  Abs. : Abs  SaturateOnIntegerOverflow=off
  Check Vertical Friction : Product  RndMeth=Zero
  FixPt Relational Operator : RelationalOperator  Operator=>  OutDataTypeStr=boolean  ZeroCross=off  InputSameDT=off
  Gain3 : Gain  Gain=GC.k_gx
  Gain4 : Gain  Gain=1/v.gx_max
  Memory : Memory
  Mux1 : Mux  Inputs=2
  Positive : simulink/Logic and Bit Operations/Compare To Zero  relop=>  OutDataTypeStr=boolean
  Positive1 : simulink/Logic and Bit Operations/Compare To Zero  relop=>  OutDataTypeStr=boolean
  Sum : Sum  Inputs=-+
  Sum2 : Sum  Inputs=-+|
  X-Axis Stiction Force2 : Fcn  Expr=-u(1) * (1+sgn(u(1))*u(2)) * ( (1+sgn(u(1))*u(2))>0)
  stiction limit force : Gain  Gain=mu.stick
  F_Stick [N] : Outport  OutputWhenDisabled=reset  InitialOutput=0  VectorParamsAs1DForOutWhenUnconnected=off
      settings: AttributesFormatString=when disabled: %<OutputWhenDisabled>\ninitial: %<InitialOutput>
  Sliding! : Outport  Port=2  OutputWhenDisabled=reset  InitialOutput=0  VectorParamsAs1DForOutWhenUnconnected=off
      settings: AttributesFormatString=when disabled: %<OutputWhenDisabled>\ninitial: %<InitialOutput>
  wires:
  F_Normal [N]/1 -> stiction limit force/1, Positive1/1
  Sum2/1 -> Gain3/1  "dx"
  pos [m]/1 -> Sum2/2
  posFP [m]/1 -> Sum2/1
  vel [m/s]/1 -> Gain4/1
  Sum/1 -> Positive/1
  Memory/1 -> FixPt Relational Operator/2
  Positive/1 -> FixPt Relational Operator/1, Memory/1
  Abs./1 -> Sum/2
  Mux1/1 -> X-Axis Stiction Force2/1
  Gain3/1 -> Mux1/1
  Gain4/1 -> Mux1/2
  FixPt Relational Operator/1 -> Sliding!/1
  Abs/1 -> Sum/1
  stiction limit force/1 -> Abs/1
  Positive1/1 -> Check Vertical Friction/2
  Check Vertical Friction/1 -> F_Stick [N]/1, Abs./1
  X-Axis Stiction Force2/1 -> Check Vertical Friction/1

== system JenaFox_NCm/JenaFox Model/GCM Right/Ground Friction Model/Friction Switch ==
  note: Static/Kinetic Friction Switch
  Slide! : Inport
  Stick! : Inport  Port=2
  Memory : Memory
  S-R Flip-Flop : simulink_extras/Flip Flops/S-R Flip-Flop  initial_condition=1
  Terminator : Terminator
  Stiction : Outport  VectorParamsAs1DForOutWhenUnconnected=off
  wires:
  S-R Flip-Flop/1 -> Memory/1
  S-R Flip-Flop/2 -> Terminator/1
  Stick!/1 -> S-R Flip-Flop/1
  Slide!/1 -> S-R Flip-Flop/2
  Memory/1 -> Stiction/1
